simulink model "Motor_Cable_verification"  (R2019b)
settings: Solver=VariableStepAuto  StartTime=0.0  StopTime=10.0  RelTol=1e-3
values from neighbouring files (symbols this model uses):
  S = 8/1000    (= 0.008)    [parameters.m]
  theta_m = zeros(2*N,1)    [parameters.m]
settings Model: Creator=zceeash  LastModifiedBy=zceeash

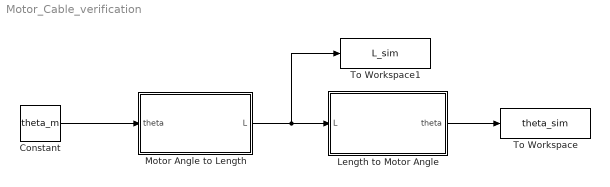
== system Motor_Cable_verification ==
  Constant : Constant  Value=theta_m
  Length to Motor Angle : Subsystem
  Motor Angle to Length : Subsystem
  To Workspace : ToWorkspace  VariableName=theta_sim  SaveFormat=Timeseries  SampleTime=-1
  To Workspace1 : ToWorkspace  VariableName=L_sim  SaveFormat=Timeseries  SampleTime=-1
  wires:
  Motor Angle to Length/1(L) -> To Workspace1/1, Length to Motor Angle/1(L)
  Constant/1 -> Motor Angle to Length/1(theta)
  Length to Motor Angle/1(theta) -> To Workspace/1

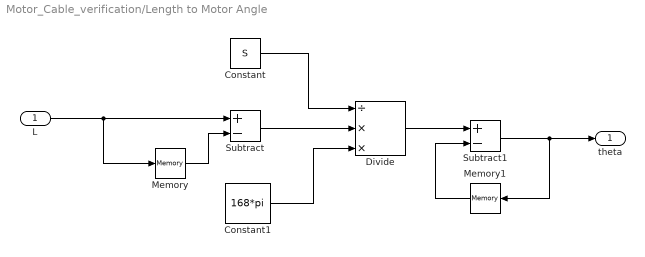
== system Motor_Cable_verification/Length to Motor Angle ==
  L : Inport
  Constant : Constant  Value=S
  Constant1 : Constant  Value=168*pi
  Divide : Product  Inputs=/**
  Memory : Memory
  Memory1 : Memory
  Subtract : Sum  Inputs=+-
  Subtract1 : Sum  Inputs=+-
  theta : Outport
  wires:
  Constant/1 -> Divide/1
  Constant1/1 -> Divide/3
  Memory/1 -> Subtract/2
  Memory1/1 -> Subtract1/2
  Subtract1/1 -> Memory1/1, theta/1
  Subtract/1 -> Divide/2
  Divide/1 -> Subtract1/1
  L/1 -> Subtract/1, Memory/1

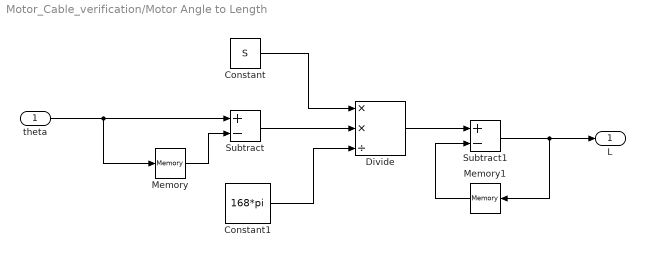
== system Motor_Cable_verification/Motor Angle to Length ==
  theta : Inport
  Constant : Constant  Value=S
  Constant1 : Constant  Value=168*pi
  Divide : Product  Inputs=**/
  Memory : Memory
  Memory1 : Memory
  Subtract : Sum  Inputs=+-
  Subtract1 : Sum  Inputs=+-
  L : Outport
  wires:
  theta/1 -> Subtract/1, Memory/1
  Subtract/1 -> Divide/2
  Memory/1 -> Subtract/2
  Divide/1 -> Subtract1/1
  Memory1/1 -> Subtract1/2
  Subtract1/1 -> Memory1/1, L/1
  Constant/1 -> Divide/1
  Constant1/1 -> Divide/3
